simulink model "Time_model_wI"  (R2023b)
settings: Solver=VariableStepAuto  StartTime=10  StopTime=40  FixedStep=0.5  RelTol=1e-3
settings Model: PacingRate=0.800000  Creator=20181234  LastModifiedBy=20181234
settings SolverCC: AlgebraicLoopSolver=TrustRegion
settings OptimizationCC: ReuseModelBlockBuffer=off
settings DebuggingCC: UnconnectedInputMsg=warning  UnconnectedOutputMsg=warning  UnconnectedLineMsg=warning
settings ModelReferenceCC: EnableRefExpFcnMdlSchedulingChecks=on
settings RTWCC: DLArmComputeVersion=19.05

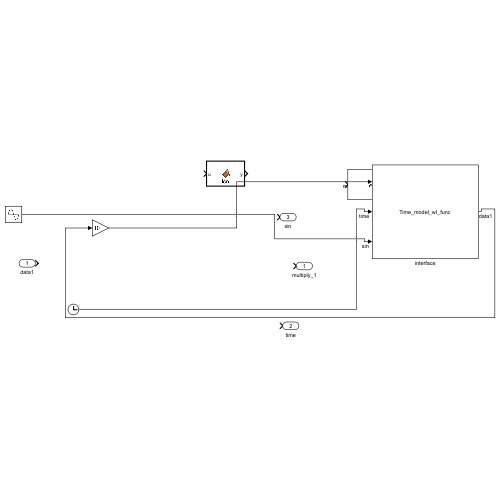
[thumbnail: Simulink's stored preview of the top-level diagram]
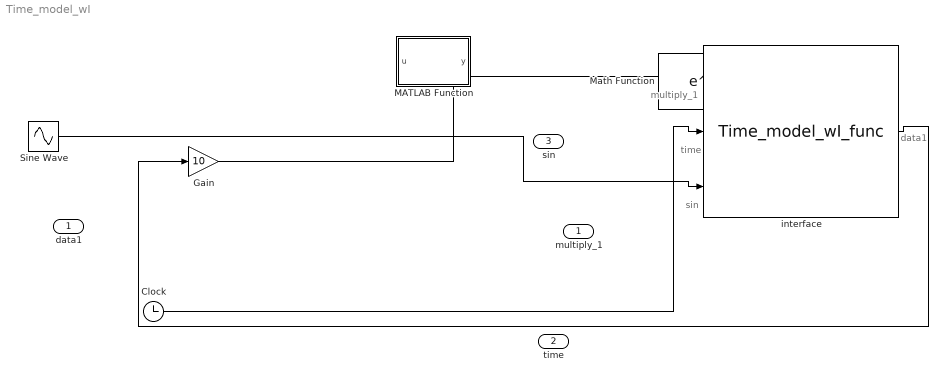
== system Time_model_wI ==
  note: multiply_1
  note: time
  note: sin
  note: data1
  data1 : Inport
  Clock : Clock
  Gain : Gain  Gain=10
  MATLAB Function : MATLAB Function  TreatAsAtomicUnit=on
  Math Function : Math
  Sine Wave : Sin  SampleTime=0
  interface : M-S-Function  FunctionName=Time_model_wI_func
  multiply_1 : Outport
  time : Outport  Port=2
  sin : Outport  Port=3
  wires:
  Gain/1 -> interface/1
  Clock/1 -> interface/2
  interface/1 -> Gain/1
  Sine Wave/1 -> interface/3

== matlab function Time_model_wI/MATLAB Function ==
  data: u input; y output
function y = fcn(u)

y = u;
